simulink model "UserBrake_RTW"  (Simulink 8.7)
settings: Solver=ode1  SolverMode=SingleTasking  StartTime=0.0  StopTime=inf  FixedStep=0.001  RelTol=1e-3
PreLoadFcn:
  | vehicle = 'Car'; if ~length(which('cmcmd')), cmenv; end
  | UserBrake_RTW_bus
InitFcn:
  | vehicle = 'Car'; if ~length(which('cmcmd')), cmenv; end
  | UserBrake_RTW_bus
Description:
  | CarMaker Plug-in Model Target
settings Model: Creator=IPG  LastModifiedBy=IPG
settings DataIOCC: SignalLoggingSaveFormat=ModelDataLogs
settings OptimizationCC: ExpressionDepthLimit=2147483647
settings DebuggingCC: FcnCallInpInsideContextMsg=UseLocalSettings  StateNameClashWarn=warning
settings HardwareCC: TargetHWDeviceType=32-bit Generic  ProdEqTarget=off
settings RTWCC: SystemTargetFile=CarMaker.tlc  TemplateMakefile=CarMaker_unix-linux64.tmf  Description=CarMaker Plug-in Model Target
settings CodeAppCC: MaxIdLength=63
settings STFCustomTargetCC: ModelReferenceCompliant=off  GeneratePreprocessorConditionals=Disable all  MultiInstanceERTCode=on  CodeInterfacePackaging=Reusable function  CPPClassGenCompliant=on  GRTInterface=off  GenerateAllocFcn=on  SystemTargetFile=CarMaker.tlc
settings GRTTargetCC: ModelReferenceCompliant=off  ParMdlRefBuildCompliant=off  CompOptLevelCompliant=off  ConcurrentExecutionCompliant=off  CombineOutputUpdateFcns=off  MatFileLogging=off  MultiInstanceERTCode=on  CodeInterfacePackaging=Reusable function  GenerateAllocFcn=on  UseToolchainInfoCompliant=off  ExtModeMexFile=noextcomm
settings CustomProperty: DataType=string  Value=..
settings EnumStrPairs: String=Car

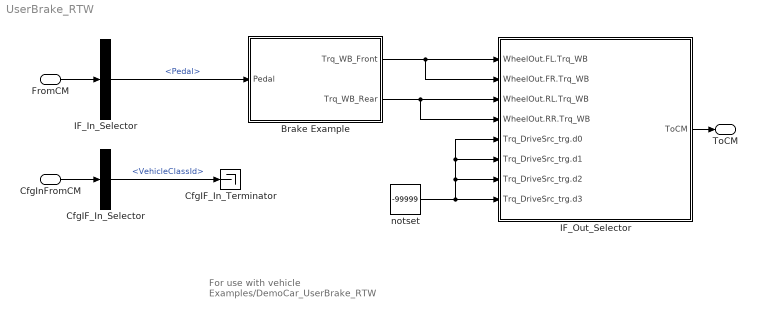
== system UserBrake_RTW ==
  note: For use with vehicle Examples/DemoCar_UserBrake_RTW
  FromCM : Inport  OutDataTypeStr=Bus: cmBrakeIn
  CfgInFromCM : Inport  Port=2  OutDataTypeStr=Bus: cmBrakeCfgIn
  Brake Example : Subsystem
  CfgIF_In_Selector : BusSelector  OutputSignals=VehicleClassId
  CfgIF_In_Terminator : Terminator
  IF_In_Selector : BusSelector  OutputSignals=Pedal
  IF_Out_Selector : Subsystem  mask(Signal Selection){}
      mask help: Signal Selection Block
      settings: OpenFcn=cmSignalSelect('SignalSelection_CB',gcb)
  notset : Constant  Value=-99999
  ToCM : Outport  OutDataTypeStr=Bus: cmBrakeOut
  wires:
  FromCM/1 -> IF_In_Selector/1
  IF_Out_Selector/1(ToCM) -> ToCM/1
  CfgInFromCM/1 -> CfgIF_In_Selector/1
  Brake Example/1(Trq_WB_Front) -> IF_Out_Selector/1(WheelOut.FL.Trq_WB), IF_Out_Selector/2(WheelOut.FR.Trq_WB)
  Brake Example/2(Trq_WB_Rear) -> IF_Out_Selector/4(WheelOut.RR.Trq_WB), IF_Out_Selector/3(WheelOut.RL.Trq_WB)
  CfgIF_In_Selector/1 -> CfgIF_In_Terminator/1  "<VehicleClassId>"
  IF_In_Selector/1 -> Brake Example/1(Pedal)  "<Pedal>"
  notset/1 -> IF_Out_Selector/7(Trq_DriveSrc_trg.d2), IF_Out_Selector/5(Trq_DriveSrc_trg.d0), IF_Out_Selector/6(Trq_DriveSrc_trg.d1), IF_Out_Selector/8(Trq_DriveSrc_trg.d3)

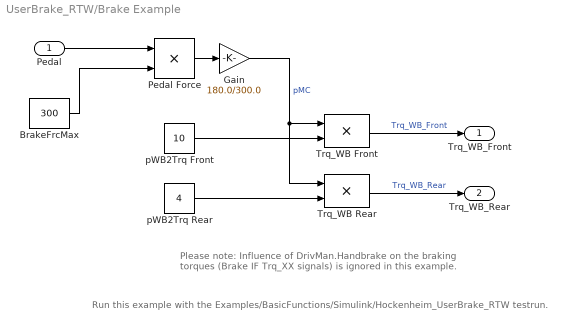
== system UserBrake_RTW/Brake Example ==
  note: Run this example with the Examples/BasicFunctions/Simulink/Hockenheim_UserBrake_RTW testrun.
  note: Please note: Influence of DrivMan.Handbrake on the braking
      | torques (Brake IF Trq_XX signals) is ignored in this example.
  Pedal : Inport
  BrakeFrcMax : Constant  Value=300
  Gain : Gain  Gain=180.0/300.0  SaturateOnIntegerOverflow=on  OutDataTypeStr=Inherit: Same as input  ParamDataTypeStr=Inherit: Same as input
  Pedal Force : Product  SaturateOnIntegerOverflow=on  InputSameDT=on  OutDataTypeStr=Inherit: Same as first input
  Trq_WB Front : Product  SaturateOnIntegerOverflow=on  InputSameDT=on  OutDataTypeStr=Inherit: Same as first input
  Trq_WB Rear : Product  SaturateOnIntegerOverflow=on  InputSameDT=on  OutDataTypeStr=Inherit: Same as first input
  pWB2Trq Front : Constant  Value=10
  pWB2Trq Rear : Constant  Value=4
  Trq_WB_Front : Outport
  Trq_WB_Rear : Outport  Port=2
  wires:
  Trq_WB Rear/1 -> Trq_WB_Rear/1  "Trq_WB_Rear"
  Trq_WB Front/1 -> Trq_WB_Front/1  "Trq_WB_Front"
  Pedal/1 -> Pedal Force/1
  BrakeFrcMax/1 -> Pedal Force/2
  Gain/1 -> Trq_WB Rear/1, Trq_WB Front/1  "pMC"
  pWB2Trq Front/1 -> Trq_WB Front/2
  pWB2Trq Rear/1 -> Trq_WB Rear/2
  Pedal Force/1 -> Gain/1

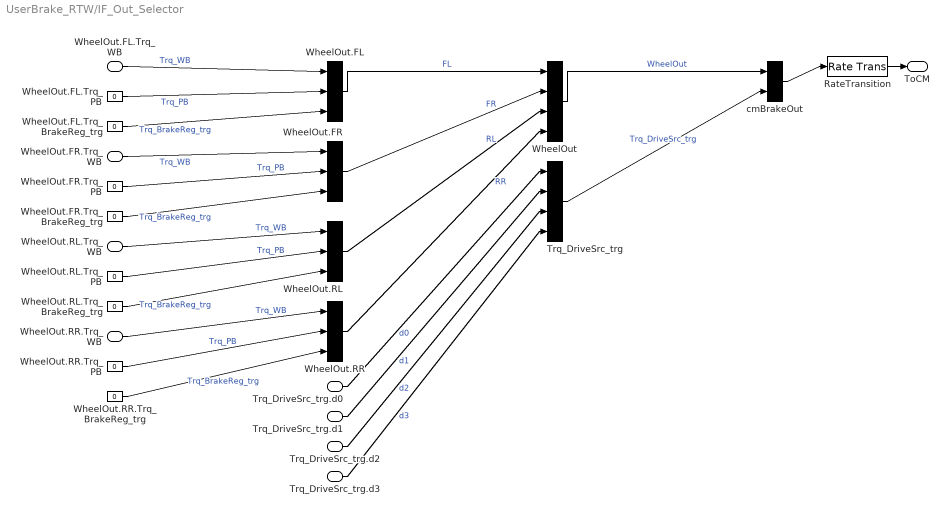
== system UserBrake_RTW/IF_Out_Selector ==
  WheelOut.FL.Trq_WB : Inport
  WheelOut.FR.Trq_WB : Inport  Port=2
  WheelOut.RL.Trq_WB : Inport  Port=3
  WheelOut.RR.Trq_WB : Inport  Port=4
  Trq_DriveSrc_trg.d0 : Inport  Port=5
  Trq_DriveSrc_trg.d1 : Inport  Port=6
  Trq_DriveSrc_trg.d2 : Inport  Port=7
  Trq_DriveSrc_trg.d3 : Inport  Port=8
  RateTransition : RateTransition  OutPortSampleTime=str2num(get_param(bdroot,'FixedStep'))
  Trq_DriveSrc_trg : BusCreator  Inputs=4
  WheelOut : BusCreator  Inputs=4
  WheelOut.FL : BusCreator  Inputs=3
  WheelOut.FL.Trq_BrakeReg_trg : Constant  Value=0
  WheelOut.FL.Trq_PB : Constant  Value=0
  WheelOut.FR : BusCreator  Inputs=3
  WheelOut.FR.Trq_BrakeReg_trg : Constant  Value=0
  WheelOut.FR.Trq_PB : Constant  Value=0
  WheelOut.RL : BusCreator  Inputs=3
  WheelOut.RL.Trq_BrakeReg_trg : Constant  Value=0
  WheelOut.RL.Trq_PB : Constant  Value=0
  WheelOut.RR : BusCreator  Inputs=3
  WheelOut.RR.Trq_BrakeReg_trg : Constant  Value=0
  WheelOut.RR.Trq_PB : Constant  Value=0
  cmBrakeOut : BusCreator  Inputs=2
  ToCM : Outport
  wires:
  RateTransition/1 -> ToCM/1
  cmBrakeOut/1 -> RateTransition/1
  WheelOut/1 -> cmBrakeOut/1  "WheelOut"
  WheelOut.FL/1 -> WheelOut/1  "FL"
  WheelOut.FL.Trq_PB/1 -> WheelOut.FL/2  "Trq_PB"
  WheelOut.FL.Trq_BrakeReg_trg/1 -> WheelOut.FL/3  "Trq_BrakeReg_trg"
  WheelOut.FR/1 -> WheelOut/2  "FR"
  WheelOut.FR.Trq_PB/1 -> WheelOut.FR/2  "Trq_PB"
  WheelOut.FR.Trq_BrakeReg_trg/1 -> WheelOut.FR/3  "Trq_BrakeReg_trg"
  WheelOut.RL/1 -> WheelOut/3  "RL"
  WheelOut.RL.Trq_PB/1 -> WheelOut.RL/2  "Trq_PB"
  WheelOut.RL.Trq_BrakeReg_trg/1 -> WheelOut.RL/3  "Trq_BrakeReg_trg"
  WheelOut.RR/1 -> WheelOut/4  "RR"
  WheelOut.RR.Trq_PB/1 -> WheelOut.RR/2  "Trq_PB"
  WheelOut.RR.Trq_BrakeReg_trg/1 -> WheelOut.RR/3  "Trq_BrakeReg_trg"
  Trq_DriveSrc_trg/1 -> cmBrakeOut/2  "Trq_DriveSrc_trg"
  WheelOut.FL.Trq_WB/1 -> WheelOut.FL/1  "Trq_WB"
  WheelOut.FR.Trq_WB/1 -> WheelOut.FR/1  "Trq_WB"
  WheelOut.RL.Trq_WB/1 -> WheelOut.RL/1  "Trq_WB"
  WheelOut.RR.Trq_WB/1 -> WheelOut.RR/1  "Trq_WB"
  Trq_DriveSrc_trg.d0/1 -> Trq_DriveSrc_trg/1  "d0"
  Trq_DriveSrc_trg.d1/1 -> Trq_DriveSrc_trg/2  "d1"
  Trq_DriveSrc_trg.d2/1 -> Trq_DriveSrc_trg/3  "d2"
  Trq_DriveSrc_trg.d3/1 -> Trq_DriveSrc_trg/4  "d3"
